simulink model "HDLLTE"  (R2017b)
settings: Solver=FixedStepDiscrete  StartTime=0.0  StopTime=simParams.stopTime  RelTol=1e-3
InitFcn:
  | simParams = hdlcoder_lteofdm_modDetectref_init;
  | simParams = hdlcoder_lteofdm_modDetecthdl_init(simParams);
StopFcn:
  | hdlcoder_lteofdm_modDetect_analyze;
undefined symbols (not defined in the file): fft_size
libraries: hdlsllib x29, simulink x22, simulink_need_slupdate x13, dspxfrm3 x2, commchan3 x1, dspmlti4 x1, commrflib2 x1, hdlcodermisc x1, dspsigops x1, dspmathops x1, dspsrcs4 x1
(part 2 of 3)

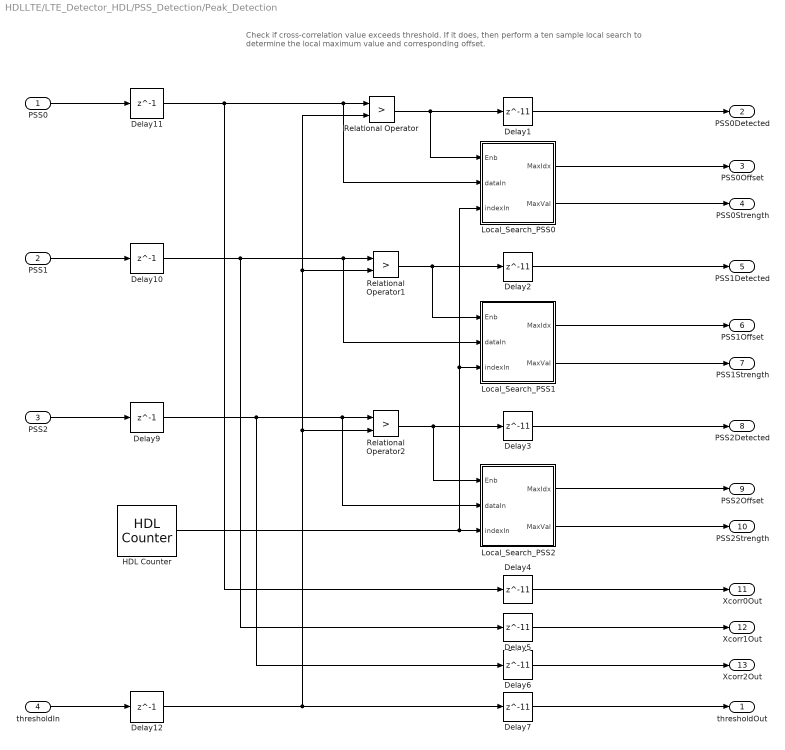
== system HDLLTE/LTE_Detector_HDL/PSS_Detection/Peak_Detection ==
  note: Check if cross-correlation value exceeds threshold. If it does, then perform a ten sample local search to determine the local maximum value and corresponding offset.
  PSS0 : Inport
  PSS1 : Inport  Port=2
  PSS2 : Inport  Port=3
  thresholdIn : Inport  Port=4
  Delay{1..7} (7 alike) : Delay  DelayLength=11  InitialCondition=0
  Delay{9..12} (4 alike) : Delay  DelayLength=1  InitialCondition=0  UseCircularBuffer=on
  HDL Counter : hdlsllib/Sources/HDL Counter  CountType=Count limited  CountInit=0  CountStep=1  CountMax=19199  CountFromType=Initial value  CountFrom=0  CountResetPort=off  CountLoadPort=off  CountEnbPort=off  CountDirPort=off  CountDataType=Unsigned  CountWordLen=ceil(log2(19199))  CountFracLen=0  CountSampTime=simParams.TsRx
      settings: SourceProductBaseCode=HD
  Local_Search_PSS0 : Subsystem
  Local_Search_PSS1 : Subsystem
  Local_Search_PSS2 : Subsystem
  Relational Operator : RelationalOperator  Operator=>  OutDataTypeStr=boolean  RndMeth=Nearest
  Relational Operator1 : RelationalOperator  Operator=>  OutDataTypeStr=boolean  RndMeth=Nearest
  Relational Operator2 : RelationalOperator  Operator=>  OutDataTypeStr=boolean  RndMeth=Nearest
  thresholdOut : Outport  InitialOutput=0
  PSS0Detected : Outport  Port=2
  PSS0Offset : Outport  Port=3
  PSS0Strength : Outport  Port=4
  PSS1Detected : Outport  Port=5
  PSS1Offset : Outport  Port=6
  PSS1Strength : Outport  Port=7
  PSS2Detected : Outport  Port=8
  PSS2Offset : Outport  Port=9
  PSS2Strength : Outport  Port=10
  Xcorr0Out : Outport  Port=11  InitialOutput=0
  Xcorr1Out : Outport  Port=12  InitialOutput=0
  Xcorr2Out : Outport  Port=13  InitialOutput=0
  wires:
  thresholdIn/1 -> Delay12/1
  PSS2/1 -> Delay9/1
  PSS1/1 -> Delay10/1
  Relational Operator/1 -> Delay1/1, Local_Search_PSS0/1(Enb)
  Relational Operator1/1 -> Local_Search_PSS1/1(Enb), Delay2/1
  Relational Operator2/1 -> Local_Search_PSS2/1(Enb), Delay3/1
  PSS0/1 -> Delay11/1
  Local_Search_PSS0/1(MaxIdx) -> PSS0Offset/1
  Local_Search_PSS0/2(MaxVal) -> PSS0Strength/1
  Local_Search_PSS1/1(MaxIdx) -> PSS1Offset/1
  Local_Search_PSS1/2(MaxVal) -> PSS1Strength/1
  Local_Search_PSS2/1(MaxIdx) -> PSS2Offset/1
  Local_Search_PSS2/2(MaxVal) -> PSS2Strength/1
  Delay1/1 -> PSS0Detected/1
  Delay2/1 -> PSS1Detected/1
  Delay3/1 -> PSS2Detected/1
  Delay4/1 -> Xcorr0Out/1
  Delay5/1 -> Xcorr1Out/1
  Delay6/1 -> Xcorr2Out/1
  Delay7/1 -> thresholdOut/1
  HDL Counter/1 -> Local_Search_PSS2/3(indexIn), Local_Search_PSS1/3(indexIn), Local_Search_PSS0/3(indexIn)
  Delay9/1 -> Delay6/1, Local_Search_PSS2/2(dataIn), Relational Operator2/1
  Delay10/1 -> Delay5/1, Local_Search_PSS1/2(dataIn), Relational Operator1/1
  Delay11/1 -> Local_Search_PSS0/2(dataIn), Relational Operator/1, Delay4/1
  Delay12/1 -> Relational Operator/2, Relational Operator1/2, Relational Operator2/2, Delay7/1

== system HDLLTE/LTE_Detector_HDL/SSS_Detection/SSS_Dot_Product ==
  note: Accumulate
  note: Reset register after all 63 samples have been processed
  note: Only final sample from accumulator is valid
  note: Multiply dataIn by seqIn:
      | since seqIn is always either -1 or 1, use a gain of -1 and a switch to invert dataIn when seqIn = -1.
  dataIn : Inport
  validIn : Inport  Port=2
  seqIn : Inport  Port=3
  reset : Inport  Port=4
  Add : Sum  OutDataTypeStr=Inherit: Same as first input
  Compare To Zero1 : simulink/Logic and Bit Operations/Compare To Zero  relop=<  OutDataTypeStr=boolean
  Data Type Conversion : DataTypeConversion  OutDataTypeStr=fixdt(1,24,10)
  Data Type Conversion1 : DataTypeConversion  OutDataTypeStr=fixdt(1,18,4)  RndMeth=Round
  Delay Reset : Subsystem
  Delay1 : Delay  DelayLength=1  InitialCondition=0
  Delay2 : Delay  DelayLength=4  InitialCondition=0
  Delay3 : Delay  InitialCondition=0
  Delay5 : Delay  DelayLength=1  InitialCondition=0
  Gain : Gain  Gain=-1  OutDataTypeStr=Inherit: Same as input
  Magnitude Squared 0 : Subsystem
  real1 : Switch  Criteria=u2 ~= 0
  validOut : Outport  InitialOutput=0
  SSSDotProd : Outport  Port=2  InitialOutput=0
  wires:
  Delay2/1 -> validOut/1
  Delay3/1 -> Delay2/1, Delay Reset/3(R)
  Delay5/1 -> Delay Reset/2(E)
  Add/1 -> Delay Reset/1(u)
  validIn/1 -> Delay5/1
  Delay1/1 -> Data Type Conversion/1
  Magnitude Squared 0/1(Magnitude^2) -> SSSDotProd/1
  reset/1 -> Delay3/1
  Delay Reset/1(y) -> Add/2, Data Type Conversion1/1
  Data Type Conversion/1 -> Add/1
  real1/1 -> Delay1/1
  dataIn/1 -> Gain/1, real1/3
  Gain/1 -> real1/1
  seqIn/1 -> Compare To Zero1/1
  Compare To Zero1/1 -> real1/2
  Data Type Conversion1/1 -> Magnitude Squared 0/1(dataIn)

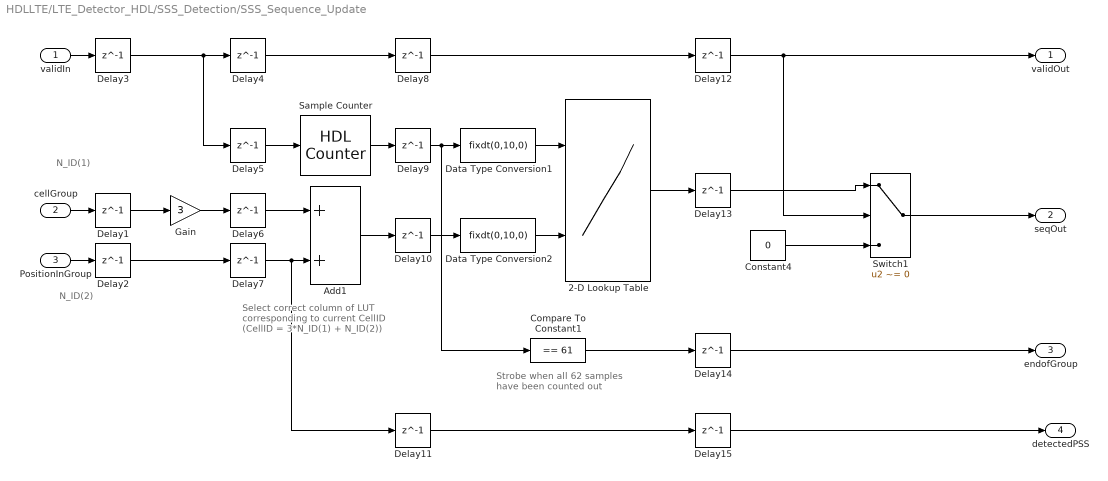
== system HDLLTE/LTE_Detector_HDL/SSS_Detection/SSS_Sequence_Update ==
  note: N_ID(2)
  note: Select correct column of LUT
      | corresponding to current CellID
      | (CellID = 3*N_ID(1) + N_ID(2))
  note: N_ID(1)
  note: Strobe when all 62 samples
      | have been counted out
  validIn : Inport
  cellGroup : Inport  Port=2
  PositionInGroup : Inport  Port=3
  2-D Lookup Table : Lookup_n-D  BreakpointsForDimension1=[0:size(simParams.possibleSSS,1)-1]  BreakpointsForDimension2=[0:size(simParams.possibleSSS,2)-1]  IndexSearchMethod=Evenly spaced points  Table=real(simParams.possibleSSS)  TableDataTypeStr=fixdt(1,2,0)  InterpMethod=Flat  DiagnosticForOutOfRangeInput=Error  InternalRulePriority=Speed  OutDataTypeStr=fixdt(1,2,0)  RndMeth=Simplest  InputSameDT=on
  Add1 : Sum  OutDataTypeStr=Inherit: Same as first input
  Compare To Constant1 : simulink/Logic and Bit Operations/Compare To Constant  relop===  const=61  OutDataTypeStr=boolean
  Constant4 : Constant  Value=0  OutDataTypeStr=fixdt(1,2,0)  SampleTime=simParams.TsRx
  Data Type Conversion1 : DataTypeConversion  OutDataTypeStr=fixdt(0,10,0)
  Data Type Conversion2 : DataTypeConversion  OutDataTypeStr=fixdt(0,10,0)
  Delay{1..15} (15 alike) : Delay  DelayLength=1  InitialCondition=0
  Gain : Gain  Gain=3  OutDataTypeStr=fixdt(0,10,0)
  Sample Counter : hdlsllib/Sources/HDL Counter  CountType=Count limited  CountInit=0  CountStep=1  CountMax=61  CountFromType=Initial value  CountFrom=0  CountResetPort=off  CountLoadPort=off  CountEnbPort=on  CountDirPort=off  CountDataType=Unsigned  CountWordLen=ceil(log2(61))  CountFracLen=0  CountSampTime=1
      settings: SourceProductBaseCode=HD
  Switch1 : Switch  Criteria=u2 ~= 0
  validOut : Outport  InitialOutput=0
  seqOut : Outport  Port=2  InitialOutput=0
  endofGroup : Outport  Port=3  InitialOutput=0
  detectedPSS : Outport  Port=4  InitialOutput=0
  wires:
  Constant4/1 -> Switch1/3
  Data Type Conversion1/1 -> 2-D Lookup Table/1
  Data Type Conversion2/1 -> 2-D Lookup Table/2
  2-D Lookup Table/1 -> Delay13/1
  Compare To Constant1/1 -> Delay14/1
  cellGroup/1 -> Delay1/1
  Gain/1 -> Delay6/1
  validIn/1 -> Delay3/1
  Sample Counter/1 -> Delay9/1
  Add1/1 -> Delay10/1
  PositionInGroup/1 -> Delay2/1
  Delay3/1 -> Delay4/1, Delay5/1
  Delay1/1 -> Gain/1
  Delay2/1 -> Delay7/1
  Delay4/1 -> Delay8/1
  Delay5/1 -> Sample Counter/1
  Delay6/1 -> Add1/1
  Delay7/1 -> Delay11/1, Add1/2
  Delay8/1 -> Delay12/1
  Delay9/1 -> Data Type Conversion1/1, Compare To Constant1/1
  Delay10/1 -> Data Type Conversion2/1
  Delay11/1 -> Delay15/1
  Delay12/1 -> validOut/1, Switch1/2
  Delay13/1 -> Switch1/1
  Switch1/1 -> seqOut/1
  Delay14/1 -> endofGroup/1
  Delay15/1 -> detectedPSS/1

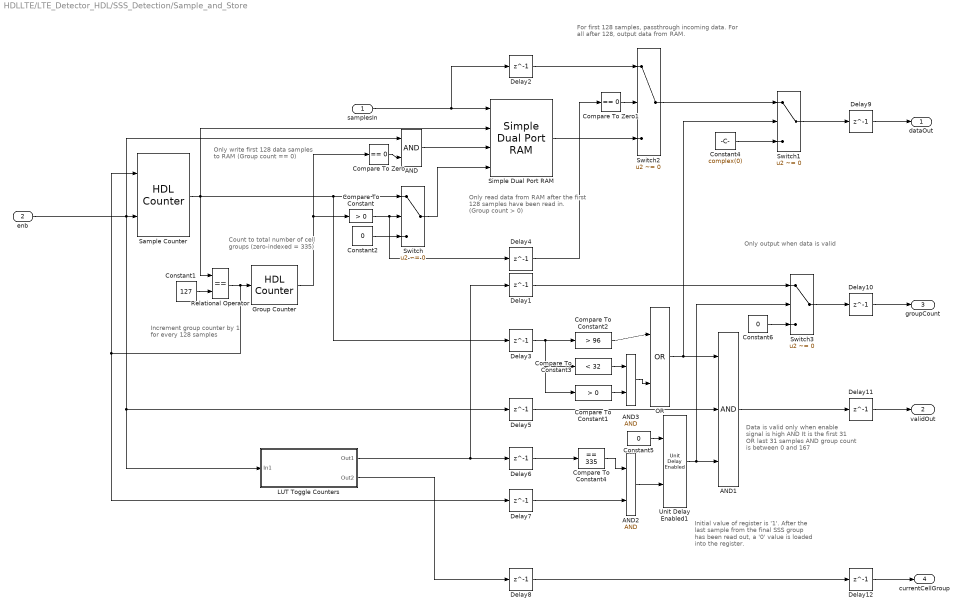
== system HDLLTE/LTE_Detector_HDL/SSS_Detection/Sample_and_Store ==
  note: Count to total number of
      | cell groups
      | (zero-indexed = 335)
  note: For first 128 samples, passthrough incoming data.
      | For all after 128, output data from RAM.
  note: Data is valid only when enable
      | signal is high AND It is the first
      | 31 OR last 31 samples AND
      | group count is between 0 and 167
  note: Only read data from RAM after the
      | first 128 samples have been read in.
      | (Group count > 0)
  note: Only write first 128 data samples
      | to RAM (Group count == 0)
  note: Increment group counter by 1
      | for every 128 samples
  note: Initial value of register is '1'.
      | After the last sample from the
      | final SSS group has been read out,
      | a '0' value is loaded into the register.
  note: Only output when data is valid
  samplesIn : Inport
  enb : Inport  Port=2
  AND : Logic  IconShape=distinctive  AllPortsSameDT=off  OutDataTypeStr=boolean
  AND1 : Logic  Inputs=3  IconShape=distinctive  AllPortsSameDT=off  OutDataTypeStr=boolean
  AND2 : Logic  IconShape=distinctive  AllPortsSameDT=off  OutDataTypeStr=boolean
  AND3 : Logic  IconShape=distinctive  AllPortsSameDT=off  OutDataTypeStr=boolean
  Compare To Constant : simulink/Logic and Bit Operations/Compare To Constant  relop=>  const=0  OutDataTypeStr=boolean
  Compare To Constant1 : simulink/Logic and Bit Operations/Compare To Constant  relop=>  const=0  OutDataTypeStr=boolean
  Compare To Constant2 : simulink/Logic and Bit Operations/Compare To Constant  relop=>  const=96  OutDataTypeStr=boolean
  Compare To Constant3 : simulink/Logic and Bit Operations/Compare To Constant  relop=<  const=32  OutDataTypeStr=boolean
  Compare To Constant4 : simulink/Logic and Bit Operations/Compare To Constant  relop===  const=335  OutDataTypeStr=boolean
  Compare To Zero : simulink/Logic and Bit Operations/Compare To Zero  relop===  OutDataTypeStr=boolean
  Compare To Zero1 : simulink/Logic and Bit Operations/Compare To Zero  relop===  OutDataTypeStr=boolean
  Constant1 : Constant  Value=127  OutDataTypeStr=fixdt(0,8,0)  SampleTime=simParams.TsRx
  Constant2 : Constant  Value=0  OutDataTypeStr=fixdt(0,7,0)  SampleTime=simParams.TsRx
  Constant4 : Constant  Value=complex(0)  OutDataTypeStr=Inherit: Inherit via back propagation  SampleTime=simParams.TsRx
  Constant5 : Constant  Value=0  OutDataTypeStr=boolean  SampleTime=simParams.TsRx
  Constant6 : Constant  Value=0  OutDataTypeStr=fixdt(0,9,0)  SampleTime=simParams.TsRx
  Delay{1..12} (12 alike) : Delay  DelayLength=1  InitialCondition=0
  Group Counter : hdlsllib/Sources/HDL Counter  CountType=Count limited  CountInit=0  CountStep=1  CountMax=335  CountFromType=Initial value  CountFrom=0  CountResetPort=off  CountLoadPort=off  CountEnbPort=on  CountDirPort=off  CountDataType=Unsigned  CountWordLen=ceil(log2(335))  CountFracLen=0  CountSampTime=1
      settings: SourceProductBaseCode=HD
  LUT Toggle Counters : Subsystem
  OR : Logic  Operator=OR  IconShape=distinctive  AllPortsSameDT=off  OutDataTypeStr=boolean
  Relational Operator : RelationalOperator  Operator===  OutDataTypeStr=boolean  RndMeth=Nearest
  Sample Counter : hdlsllib/Sources/HDL Counter  CountType=Count limited  CountInit=0  CountStep=1  CountMax=127  CountFromType=Initial value  CountFrom=0  CountResetPort=on  CountLoadPort=off  CountEnbPort=on  CountDirPort=off  CountDataType=Unsigned  CountWordLen=log2(128)  CountFracLen=0  CountSampTime=1
      settings: SourceProductBaseCode=HD
  Simple Dual Port RAM : hdlsllib/HDL RAMs/Simple Dual Port RAM  ram_size=7
      settings: SourceProductName=HDL Coder  SourceProductBaseCode=HD
  Switch : Switch  Criteria=u2 ~= 0
  Switch1 : Switch  Criteria=u2 ~= 0  InputSameDT=on
  Switch2 : Switch  Criteria=u2 ~= 0
  Switch3 : Switch  Criteria=u2 ~= 0
  Unit Delay Enabled1 : simulink_need_slupdate/Unit Delay Enabled  vinit=1  tsamp=-1
      settings: SourceProductName=Simulink  SourceProductBaseCode=SL
  dataOut : Outport
  validOut : Outport  Port=2
  groupCount : Outport  Port=3
  currentCellGroup : Outport  Port=4
  wires:
  Compare To Constant1/1 -> AND3/2
  Compare To Constant3/1 -> AND3/1
  AND3/1 -> OR/2
  Constant6/1 -> Switch3/3
  Delay7/1 -> AND2/2
  Unit Delay Enabled1/1 -> AND1/3, Switch3/2
  AND2/1 -> Unit Delay Enabled1/2
  Constant5/1 -> Unit Delay Enabled1/1
  samplesIn/1 -> Simple Dual Port RAM/1, Delay2/1
  Delay5/1 -> AND1/2
  Delay4/1 -> Compare To Zero1/1
  Delay3/1 -> Compare To Constant3/1, Compare To Constant1/1, Compare To Constant2/1
  Delay2/1 -> Switch2/1
  Switch2/1 -> Switch1/1
  Simple Dual Port RAM/1 -> Switch2/3
  Compare To Zero1/1 -> Switch2/2
  Constant4/1 -> Switch1/3
  OR/1 -> AND1/1, Switch1/2
  Compare To Constant2/1 -> OR/1
  Constant2/1 -> Switch/3
  Switch/1 -> Simple Dual Port RAM/4
  Compare To Zero/1 -> AND/2
  Compare To Constant/1 -> Switch/2, Delay4/1
  AND/1 -> Simple Dual Port RAM/3
  Constant1/1 -> Relational Operator/2
  enb/1 -> AND/1, Delay5/1, LUT Toggle Counters/1(In1), Sample Counter/2
  Group Counter/1 -> Compare To Constant/1, Compare To Zero/1
  Sample Counter/1 -> Switch/1, Delay3/1, Relational Operator/1, Simple Dual Port RAM/2
  Delay1/1 -> Switch3/1
  LUT Toggle Counters/1(Out1) -> Delay6/1, Delay1/1
  Delay6/1 -> Compare To Constant4/1
  Compare To Constant4/1 -> AND2/1
  Relational Operator/1 -> Group Counter/1, Delay7/1, Sample Counter/1
  Switch1/1 -> Delay9/1
  Switch3/1 -> Delay10/1
  AND1/1 -> Delay11/1
  LUT Toggle Counters/2(Out2) -> Delay8/1
  Delay8/1 -> Delay12/1
  Delay9/1 -> dataOut/1
  Delay10/1 -> groupCount/1
  Delay11/1 -> validOut/1
  Delay12/1 -> currentCellGroup/1

== system HDLLTE/LTE_Modulator_HDL/CP_Extension_Windowing/Compute_CP_Pass_Through_Index ==
  note: Select cyclic prefix length
  note: increment the OFDM symbol counter
      | which goes from 0 to 6
  note: Detect switch from 1 to 0 on validIn.
      | This indicates the end of an OFDM symbol
  validIn : Inport
  Add : Sum  Inputs=+-  OutDataTypeStr=uint16
  Add1 : Sum  OutDataTypeStr=uint16
  Compare To Zero : simulink/Logic and Bit Operations/Compare To Zero  relop===  OutDataTypeStr=boolean
  Constant4 : Constant  Value=simParams.nFFT  VectorParams1D=off  OutDataTypeStr=uint16  SampleTime=simParams.TsTx
  Delay1 : Delay  DelayLength=1  InitialCondition=0  InputProcessing=Columns as channels (frame based)
  Length of first CP : Constant  Value=160*(simParams.nFFT/2048)+simParams.windowing  OutDataTypeStr=uint16  SampleTime=simParams.TsTx
  Length of other CPs : Constant  Value=144*(simParams.nFFT/2048)+simParams.windowing  OutDataTypeStr=uint16  SampleTime=simParams.TsTx
  Logical Operator : Logic  IconShape=distinctive  AllPortsSameDT=off  OutDataTypeStr=boolean
  Logical Operator1 : Logic  Operator=NOT  IconShape=distinctive  AllPortsSameDT=off  OutDataTypeStr=boolean
  OFDM Symbol Counter : hdlsllib/Sources/HDL Counter  CountType=Count limited  CountInit=0  CountStep=1  CountMax=6  CountFromType=Initial value  CountFrom=0  CountResetPort=off  CountLoadPort=off  CountEnbPort=on  CountDirPort=off  CountDataType=Unsigned  CountWordLen=3  CountFracLen=0  CountSampTime=1
      settings: SourceProductBaseCode=HD
  Switch : Switch  Criteria=u2 ~= 0
  window length : Constant  Value=simParams.windowing  OutDataTypeStr=uint16  SampleTime=simParams.TsTx
  fftMinusCPandWindow : Outport
  fftMinusCP : Outport  Port=2
  wires:
  Logical Operator1/1 -> Logical Operator/1
  Length of first CP/1 -> Switch/1
  Length of other CPs/1 -> Switch/3
  OFDM Symbol Counter/1 -> Compare To Zero/1
  Compare To Zero/1 -> Switch/2
  Switch/1 -> Add/2
  validIn/1 -> Delay1/1, Logical Operator1/1
  Delay1/1 -> Logical Operator/2
  Logical Operator/1 -> OFDM Symbol Counter/1
  Constant4/1 -> Add/1
  window length/1 -> Add1/2
  Add1/1 -> fftMinusCP/1
  Add/1 -> fftMinusCPandWindow/1, Add1/1

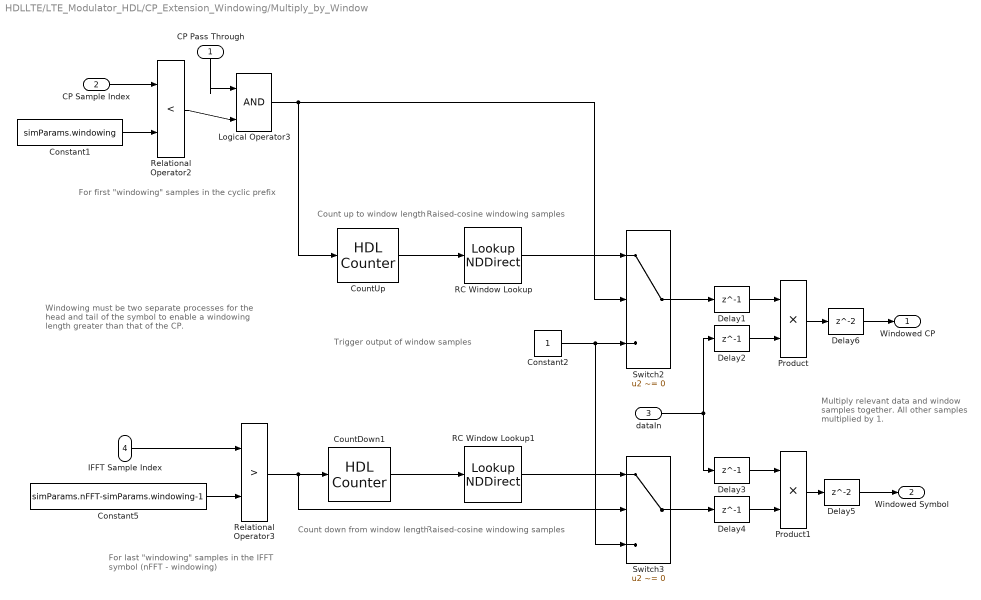
== system HDLLTE/LTE_Modulator_HDL/CP_Extension_Windowing/Multiply_by_Window ==
  note: Windowing must be two separate processes for the
      | head and tail of the symbol to enable a
      | windowing length greater than that of the CP.
  note: Multiply relevant data and window
      | samples together. All other samples
      | multiplied by 1.
  note: Count up to window length
  note: Trigger output of window samples
  note: For last "windowing" samples in the IFFT
      | symbol (nFFT - windowing)
  note: For first "windowing" samples in the cyclic prefix
  note: Raised-cosine windowing samples
  note: Count down from window length
  note: Raised-cosine windowing samples
  CP Pass Through : Inport
  CP Sample Index : Inport  Port=2
  dataIn : Inport  Port=3
  IFFT Sample Index : Inport  Port=4
  Constant1 : Constant  Value=simParams.windowing  OutDataTypeStr=uint16  SampleTime=simParams.TsTx
  Constant2 : Constant  OutDataTypeStr=fixdt(1,16,15)  SampleTime=simParams.TsTx
  Constant5 : Constant  Value=simParams.nFFT-simParams.windowing-1  OutDataTypeStr=int16  SampleTime=simParams.TsTx
  CountDown1 : hdlsllib/Sources/HDL Counter  CountType=Count limited  CountInit=simParams.LUTwindowing-1  CountStep=-1  CountMax=0  CountFromType=Initial value  CountFrom=simParams.LUTwindowing-1  CountResetPort=off  CountLoadPort=off  CountEnbPort=on  CountDirPort=off  CountDataType=Unsigned  CountWordLen=8  CountFracLen=0  CountSampTime=1
      settings: SourceProductBaseCode=HD
  CountUp : hdlsllib/Sources/HDL Counter  CountType=Count limited  CountInit=0  CountStep=1  CountMax=simParams.LUTwindowing-1  CountFromType=Initial value  CountFrom=0  CountResetPort=off  CountLoadPort=off  CountEnbPort=on  CountDirPort=off  CountDataType=Unsigned  CountWordLen=8  CountFracLen=0  CountSampTime=1
      settings: SourceProductBaseCode=HD
  Delay{1..4} (4 alike) : Delay  DelayLength=1  InitialCondition=0  InputProcessing=Columns as channels (frame based)
  Delay5 : Delay  InitialCondition=0  InputProcessing=Columns as channels (frame based)
  Delay6 : Delay  InitialCondition=0  InputProcessing=Columns as channels (frame based)
  Logical Operator3 : Logic  IconShape=distinctive  AllPortsSameDT=off  OutDataTypeStr=boolean
  Product : Product  OutDataTypeStr=Inherit: Inherit via back propagation
  Product1 : Product  OutDataTypeStr=Inherit: Inherit via back propagation
  RC Window Lookup : LookupNDDirect  NumberOfTableDimensions=1  Table=simParams.RCWindow  DiagnosticForOutOfRangeInput=Error  TableDataTypeStr=fixdt(1,16,15)
  RC Window Lookup1 : LookupNDDirect  NumberOfTableDimensions=1  Table=simParams.RCWindow  DiagnosticForOutOfRangeInput=Error  TableDataTypeStr=fixdt(1,16,15)
  Relational Operator2 : RelationalOperator  Operator=<  OutDataTypeStr=boolean  RndMeth=Nearest
  Relational Operator3 : RelationalOperator  Operator=>  OutDataTypeStr=boolean  RndMeth=Nearest
  Switch2 : Switch  Criteria=u2 ~= 0
  Switch3 : Switch  Criteria=u2 ~= 0
  Windowed CP : Outport
  Windowed Symbol : Outport  Port=2
  wires:
  Product/1 -> Delay6/1
  RC Window Lookup/1 -> Switch2/1
  CP Sample Index/1 -> Relational Operator2/1
  Constant1/1 -> Relational Operator2/2
  Relational Operator2/1 -> Logical Operator3/2
  Constant5/1 -> Relational Operator3/2
  Switch2/1 -> Delay1/1
  Product1/1 -> Delay5/1
  Switch3/1 -> Delay4/1
  Constant2/1 -> Switch3/3, Switch2/3
  IFFT Sample Index/1 -> Relational Operator3/1
  CP Pass Through/1 -> Logical Operator3/1
  RC Window Lookup1/1 -> Switch3/1
  CountUp/1 -> RC Window Lookup/1
  CountDown1/1 -> RC Window Lookup1/1
  Relational Operator3/1 -> Switch3/2, CountDown1/1
  Logical Operator3/1 -> Switch2/2, CountUp/1
  dataIn/1 -> Delay3/1, Delay2/1
  Delay1/1 -> Product/1
  Delay4/1 -> Product1/2
  Delay2/1 -> Product/2
  Delay3/1 -> Product1/1
  Delay5/1 -> Windowed Symbol/1
  Delay6/1 -> Windowed CP/1

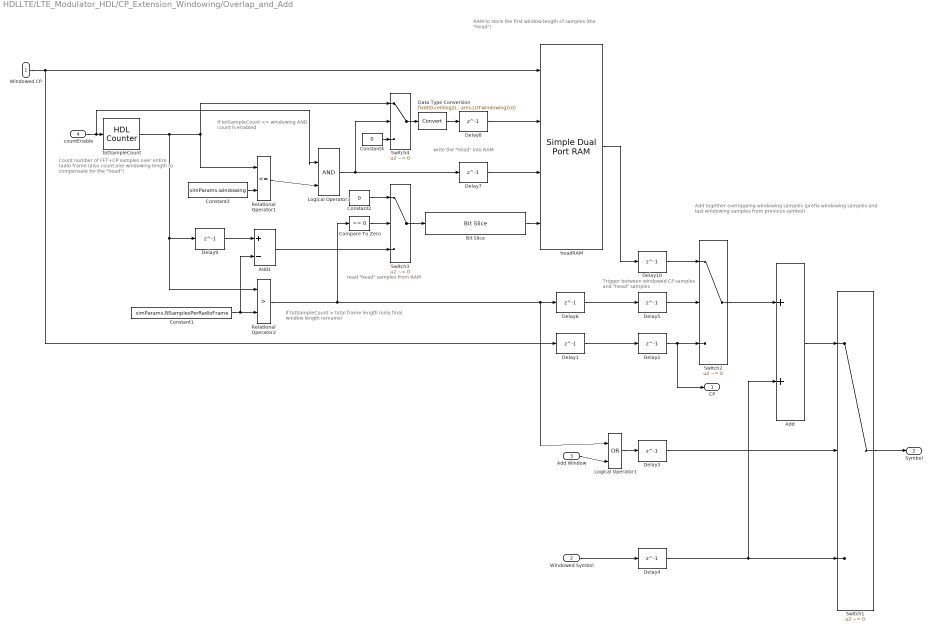
== system HDLLTE/LTE_Modulator_HDL/CP_Extension_Windowing/Overlap_and_Add ==
  note: Trigger between windowed CP samples
      | and "head" samples
  note: read "head" samples from RAM
  note: write the "head" into RAM
  note: If totSampleCount <= windowing
      | AND count is enabled
  note: if totSampleCount > total frame length
      | (only final window length remains)
  note: Add together overlapping windowing samples
      | (prefix windowing samples and last windowing samples
      | from previous symbol)
  note: RAM to store the first window length of
      | samples (the "head")
  note: Count number of FFT+CP samples
      | over entire radio frame
      | (also count one windowing length
      | to compensate for the "head")
  Windowed CP : Inport
  Windowed Symbol : Inport  Port=2
  Add Window : Inport  Port=3
  countEnable : Inport  Port=4
  Add : Sum  OutDataTypeStr=Inherit: Inherit via back propagation
  Add1 : Sum  Inputs=+-
  Bit Slice : hdlsllib/Logic and Bit Operations/Bit Slice  lidx=ceil(log2(simParams.LUTwindowing))-1  ridx=0
  Compare To Zero : simulink/Logic and Bit Operations/Compare To Zero  relop===  OutDataTypeStr=boolean
  Constant1 : Constant  Value=simParams.NSamplesPerRadioFrame  OutDataTypeStr=fixdt(0,ceil(log2(simParams.NSamplesPerRadioFrame+1)),0)  SampleTime=simParams.TsTx
  Constant2 : Constant  Value=0  OutDataTypeStr=fixdt(0,ceil(log2(simParams.LUTwindowing)),0)  SampleTime=simParams.TsTx
  Constant3 : Constant  Value=simParams.windowing  OutDataTypeStr=fixdt(0,ceil(log2(simParams.LUTwindowing)),0)  SampleTime=simParams.TsTx
  Constant4 : Constant  Value=0  OutDataTypeStr=fixdt(0,ceil(log2(simParams.LUTwindowing)),0)  SampleTime=simParams.TsTx
  Data Type Conversion : DataTypeConversion  OutDataTypeStr=fixdt(0,ceil(log2(simParams.LUTwindowing)),0)
  Delay{1..10} (10 alike) : Delay  DelayLength=1  InitialCondition=0  InputProcessing=Columns as channels (frame based)
  Logical Operator1 : Logic  Operator=OR  IconShape=distinctive  AllPortsSameDT=off  OutDataTypeStr=boolean
  Logical Operator3 : Logic  IconShape=distinctive  AllPortsSameDT=off  OutDataTypeStr=boolean
  Relational Operator1 : RelationalOperator  Operator=<=  OutDataTypeStr=boolean  RndMeth=Nearest
  Relational Operator2 : RelationalOperator  Operator=>  OutDataTypeStr=boolean  RndMeth=Nearest
  Switch{1..4} (4 alike) : Switch  Criteria=u2 ~= 0
  headRAM : hdlsllib/HDL RAMs/Simple Dual Port RAM  ram_size=ceil(log2(simParams.LUTwindowing))
      settings: SourceProductName=HDL Coder  SourceProductBaseCode=HD
  totSampleCount : hdlsllib/Sources/HDL Counter  CountType=Count limited  CountInit=0  CountStep=1  CountMax=simParams.NSamplesPerRadioFrame+simParams.windowing+1  CountFromType=Initial value  CountFrom=0  CountResetPort=off  CountLoadPort=off  CountEnbPort=on  CountDirPort=off  CountDataType=Unsigned  CountWordLen=ceil(log2(simParams.NSamplesPerRadioFrame+simParams.windowing+1))  CountFracLen=0  CountSampTime=1
      settings: SourceProductBaseCode=HD
  CP : Outport
  Symbol : Outport  Port=2
  wires:
  totSampleCount/1 -> Relational Operator2/1, Delay9/1, Switch4/1, Relational Operator1/1
  Constant3/1 -> Relational Operator1/2
  Data Type Conversion/1 -> Delay8/1
  Add/1 -> Switch1/1
  Logical Operator3/1 -> Delay7/1, Switch4/2
  Relational Operator1/1 -> Logical Operator3/2
  Logical Operator1/1 -> Delay3/1
  Delay1/1 -> Delay2/1
  Switch2/1 -> Add/1
  Add1/1 -> Switch3/3
  Switch1/1 -> Symbol/1
  Relational Operator2/1 -> Compare To Zero/1, Delay6/1, Logical Operator1/1
  Constant1/1 -> Add1/2, Relational Operator2/2
  headRAM/1 -> Delay10/1
  Constant2/1 -> Switch3/1
  Compare To Zero/1 -> Switch3/2
  Windowed Symbol/1 -> Delay4/1
  Add Window/1 -> Logical Operator1/2
  countEnable/1 -> Logical Operator3/1, totSampleCount/1
  Delay2/1 -> CP/1, Switch2/3
  Delay3/1 -> Switch1/2
  Delay4/1 -> Add/2, Switch1/3
  Delay5/1 -> Switch2/2
  Switch4/1 -> Data Type Conversion/1
  Constant4/1 -> Switch4/3
  Windowed CP/1 -> headRAM/1, Delay1/1
  Delay7/1 -> headRAM/3
  Delay8/1 -> headRAM/2
  Delay9/1 -> Add1/1
  Delay10/1 -> Switch2/1
  Switch3/1 -> Bit Slice/1
  Bit Slice/1 -> headRAM/4
  Delay6/1 -> Delay5/1

== system HDLLTE/LTE_Modulator_HDL/FFT_Shift/Compute_Read_Address ==
  note: XOR with FFT size/2 performs the fftshift on the address
      | as it flips the MSB of the index in the IFFT,
      | while XOR with FFT size flips the ping/pong
  note: select enough bits to represent 2*fft_size addresses
  note: Ping/Pong Read Address so reading from half of BlockRAM not being written to.
  note: Load Read Ptr with 0
      | and count up to fft_size  to read out data
  note: When rdEnable goes high toggle offset for Ping/Pong buffer for Read Ptr.
      | Make sure REAd and WRITE Ptr are not in same section of Ping/Pong
  note: Initial counter output is FFT size setting the counter enable to '0'.
      | When the rdEnable signal comes in, the value of 0 is loaded into
      | the counter accumulator AND output. This triggers the
      | enable signal to '1', and the counter will count up to FFT size
      | before the enable goes to '0', where the counter will remain until
      | the next load signal arrives.
  note: Alternates between outputting a '0' and '1'
      | each time the read signal is toggled high.
  rdEnable : Inport
  Bit Slice : hdlsllib/Logic and Bit Operations/Bit Slice  lidx=log2(simParams.nFFT)  ridx=0
  Bitwise Operator1 : simulink/Logic and Bit Operations/Bitwise Operator  logicop=XOR  UseBitMask=off  NumInputPorts=2  BitMask=fft_size/2  BitMaskRealWorld=Stored Integer
  Compare To Constant4 : simulink/Logic and Bit Operations/Compare To Constant  relop=<  const=simParams.nFFT  OutDataTypeStr=boolean
  Constant3 : Constant  Value=simParams.nFFT/2  OutDataTypeStr=uint16  SampleTime=simParams.TsTx
  Constant4 : Constant  Value=simParams.nFFT+simParams.nFFT/2  OutDataTypeStr=uint16  SampleTime=simParams.TsTx
  Constant6 : Constant  Value=0  OutDataTypeStr=uint16  SampleTime=simParams.TsTx
  Delay3 : Delay  DelayLength=1
  HDL Counter1 : hdlsllib/Sources/HDL Counter  CountType=Free running  CountInit=simParams.nFFT  CountStep=1  CountMax=10  CountFromType=Initial value  CountFrom=simParams.nFFT  CountResetPort=off  CountLoadPort=on  CountEnbPort=on  CountDirPort=off  CountDataType=Unsigned  CountWordLen=16  CountFracLen=0  CountSampTime=1
      settings: SourceProductBaseCode=HD
  Not : Logic  Operator=NOT  IconShape=distinctive  AllPortsSameDT=off  OutDataTypeStr=boolean
  Switch : Switch  Criteria=u2 ~= 0  Threshold=384
  Switch2 : Switch  Criteria=u2 ~= 0  Threshold=384
  rdAddr : Outport
  rdValid : Outport  Port=2
  wires:
  HDL Counter1/1 -> Compare To Constant4/1, Bitwise Operator1/1
  Compare To Constant4/1 -> HDL Counter1/3, rdValid/1
  Switch2/1 -> Delay3/1, Switch/2
  Delay3/1 -> Switch2/3, Not/1
  Not/1 -> Switch2/1
  Constant6/1 -> HDL Counter1/2
  rdEnable/1 -> HDL Counter1/1, Switch2/2
  Bit Slice/1 -> rdAddr/1
  Constant4/1 -> Switch/3
  Constant3/1 -> Switch/1
  Switch/1 -> Bitwise Operator1/2
  Bitwise Operator1/1 -> Bit Slice/1

== system HDLLTE/LTE_Modulator_HDL/OFDM_Symbol_Mapping/IFFT_Subcarrier_Counter ==
  note: Reset signal takes one clock cycle to register.
      | So reset should be triggered when count value
      | equals nFFT+CPlength-1 .
      | Hence use of nFFT-1.
  note: CP length selection.
      | 7 OFDM symbols per slot. The first symbol in the slot
      | has a longer CP length.
  note: Count until output is equal to FFT size + current CP.
      | When equal, resets bin counter and increments symbol counter.
  note: First sample values are < 0, and are reserved for the CP, and the bin count is held at nFFT . Otherwise outputs in the range of
      | 0 -> nFFT .
  Add : Sum
  Compare To Zero : simulink/Logic and Bit Operations/Compare To Zero  relop===  OutDataTypeStr=boolean
  Compare To Zero1 : simulink/Logic and Bit Operations/Compare To Zero  relop=>=  OutDataTypeStr=boolean
  FFT Size : Constant  Value=simParams.nFFT-1  OutDataTypeStr=fixdt(0,ceil(log2(simParams.nFFT)),0)  SampleTime=simParams.TsTx
  FFT Size1 : Constant  Value=simParams.nFFT  OutDataTypeStr=fixdt(0,ceil(log2(simParams.nFFT))+2,0)  SampleTime=simParams.TsTx
  HDL Counter : hdlsllib/Sources/HDL Counter  CountType=Count limited  CountInit=0  CountStep=1  CountMax=6  CountFromType=Initial value  CountFrom=0  CountResetPort=off  CountLoadPort=off  CountEnbPort=on  CountDirPort=off  CountDataType=Unsigned  CountWordLen=3  CountFracLen=0  CountSampTime=1
      settings: SourceProductBaseCode=HD
  HDL Counter2 : hdlsllib/Sources/HDL Counter  CountType=Free running  CountInit=0  CountStep=1  CountMax=6  CountFromType=Initial value  CountFrom=0  CountResetPort=on  CountLoadPort=off  CountEnbPort=off  CountDirPort=off  CountDataType=Unsigned  CountWordLen=ceil(log2(simParams.nFFT))+1  CountFracLen=0  CountSampTime=1
      settings: SourceProductBaseCode=HD
  Length of first CP : Constant  Value=160*(simParams.nFFT/2048)  OutDataTypeStr=fixdt(0,ceil(log2(simParams.nFFT)),0)  SampleTime=simParams.TsTx
  Length of other CPs : Constant  Value=144*(simParams.nFFT/2048)  OutDataTypeStr=fixdt(0,ceil(log2(simParams.nFFT)),0)  SampleTime=simParams.TsTx
  Relational Operator : RelationalOperator  Operator===  OutDataTypeStr=boolean  RndMeth=Nearest
  Subtract : Sum  Inputs=+-  OutDataTypeStr=fixdt(1,ceil(log2(simParams.nFFT))+2,0)
  Switch : Switch  Criteria=u2 ~= 0
  Switch1 : Switch  Criteria=u2 ~= 0
  IFFT subcarrier : Outport
  wires:
  Compare To Zero/1 -> Switch/2
  HDL Counter2/1 -> Subtract/1, Relational Operator/1  "Count"
  Switch/1 -> Subtract/2, Add/2
  [INCREMENT_SYMBOL] -> HDL Counter/1
  Compare To Zero1/1 -> Switch1/2
  Switch1/1 -> IFFT subcarrier/1
  Add/1 -> Relational Operator/2
  FFT Size1/1 -> Switch1/3
  Relational Operator/1 -> HDL Counter2/1, [INCREMENT_SYMBOL]
  HDL Counter/1 -> Compare To Zero/1
  Length of other CPs/1 -> Switch/3
  Subtract/1 -> Compare To Zero1/1, Switch1/1
  Length of first CP/1 -> Switch/1
  FFT Size/1 -> Add/1

== system HDLLTE/LTE_Detector_HDL/Frequency_Estimation/Cyclic_Prefix_Correlator/Moving_Average ==
  note: Use a comb filter followed by an integrator
      | to implement an efficient 9-tab moving average.
  dataIn : Inport
  Add : Sum  Inputs=-+  AccumDataTypeStr=fixdt(1,27,23)
  Add1 : Sum  AccumDataTypeStr=fixdt(1,27,23)
  Delay1 : Delay  DelayLength=8  InitialCondition=0
  Delay10 : Delay  DelayLength=1  InitialCondition=0  UseCircularBuffer=on
  Delay2 : Delay  DelayLength=1  InitialCondition=0  UseCircularBuffer=on
  Delay3 : Delay  DelayLength=1  InitialCondition=0  UseCircularBuffer=on
  Gain : Gain  Gain=1/8  OutDataTypeStr=fixdt(1,24,23)
  dataOut : Outport
  wires:
  Add/1 -> Delay10/1
  dataIn/1 -> Add/2, Delay1/1
  Delay1/1 -> Add/1
  Add1/1 -> Delay2/1
  Delay10/1 -> Add1/2
  Delay2/1 -> Gain/1, Add1/1
  Gain/1 -> Delay3/1
  Delay3/1 -> dataOut/1

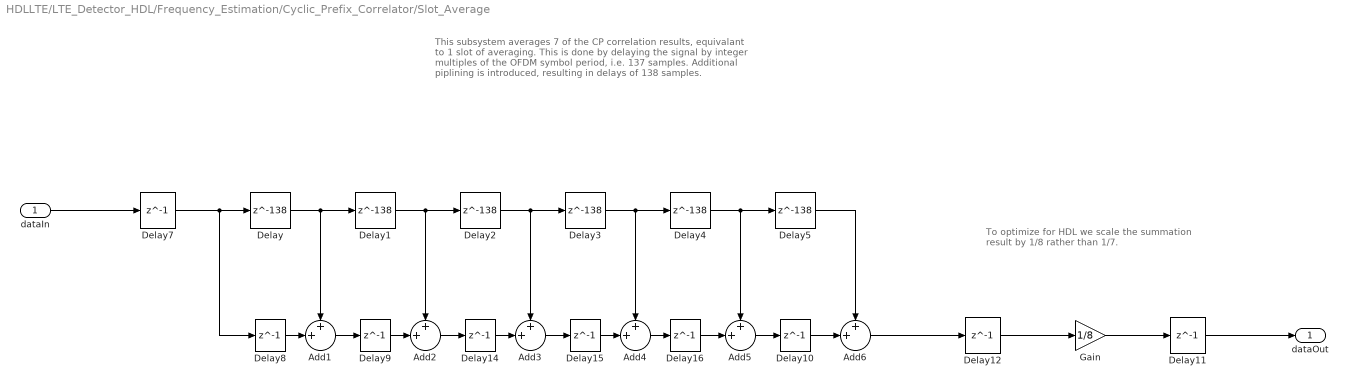
== system HDLLTE/LTE_Detector_HDL/Frequency_Estimation/Cyclic_Prefix_Correlator/Slot_Average ==
  note: This subsystem averages 7 of the CP correlation results, equivalant to 1 slot of averaging. This is done by delaying the signal by integer multiples of the OFDM symbol period, i.e. 137 samples.
      |
      | Additional piplining is introduced, resulting in delays of 138 samples.
  note: To optimize for HDL we scale the summation result by 1/8 rather than 1/7.
  dataIn : Inport
  Add1 : Sum  Inputs=++|  AccumDataTypeStr=fixdt(1,28,23)
  Add2 : Sum  Inputs=++|  AccumDataTypeStr=fixdt(1,29,23)
  Add3 : Sum  Inputs=++|  OutDataTypeStr=fixdt(1,29,23)
  Add4 : Sum  Inputs=++|  AccumDataTypeStr=fixdt(1,29,23)
  Add5 : Sum  Inputs=++|  AccumDataTypeStr=fixdt(1,30,23)
  Add6 : Sum  Inputs=++|  AccumDataTypeStr=fixdt(1,30,23)
  Delay{,1..5} (6 alike) : Delay  DelayLength=138  InitialCondition=0
  Delay{7..12,14..16} (9 alike) : Delay  DelayLength=1  InitialCondition=0  UseCircularBuffer=on
  Gain : Gain  Gain=1/8  OutDataTypeStr=fixdt(1,24,23)
  dataOut : Outport
  wires:
  Delay4/1 -> Delay5/1, Add5/1
  Delay/1 -> Delay1/1, Add1/1
  Add1/1 -> Delay9/1
  Delay1/1 -> Delay2/1, Add2/1
  Delay3/1 -> Delay4/1, Add4/1
  Delay2/1 -> Delay3/1, Add3/1
  dataIn/1 -> Delay7/1
  Add2/1 -> Delay14/1
  Add3/1 -> Delay15/1
  Add4/1 -> Delay16/1
  Add5/1 -> Delay10/1
  Delay5/1 -> Add6/1
  Add6/1 -> Delay12/1
  Delay7/1 -> Delay8/1, Delay/1
  Delay8/1 -> Add1/2
  Delay9/1 -> Add2/2
  Delay14/1 -> Add3/2
  Delay15/1 -> Add4/2
  Delay16/1 -> Add5/2
  Delay10/1 -> Add6/2
  Delay12/1 -> Gain/1
  Gain/1 -> Delay11/1
  Delay11/1 -> dataOut/1

== system HDLLTE/LTE_Detector_HDL/PSS_Detection/Cross_Correlation/Averaging_Filter ==
  datIn : Inport
  Add : Sum  Inputs=-+  AccumDataTypeStr=fixdt(1,32,23)  OutDataTypeStr=Inherit: Same as accumulator
  Add1 : Sum  AccumDataTypeStr=fixdt(1,32,23)  OutDataTypeStr=Inherit: Same as accumulator
  Delay1 : Delay  DelayLength=128  InitialCondition=0
  Delay2 : Delay  DelayLength=1  InitialCondition=0  UseCircularBuffer=on
  Delay3 : Delay  DelayLength=1  InitialCondition=0  UseCircularBuffer=on
  Gain : Gain  Gain=2^-7  OutDataTypeStr=fixdt(1,25,23)
  thresholdOut : Outport
  wires:
  Delay3/1 -> Add1/2
  Add1/1 -> Delay2/1
  Add/1 -> Delay3/1
  Delay2/1 -> Gain/1, Add1/1
  Delay1/1 -> Add/1
  datIn/1 -> Add/2, Delay1/1
  Gain/1 -> thresholdOut/1

== system HDLLTE/LTE_Detector_HDL/PSS_Detection/Cross_Correlation/Magnitude_Squared ==
  dataIn : Inport
  Add : Sum  OutDataTypeStr=Inherit: Same as accumulator
  Complex to Real-Imag : ComplexToRealImag
  Data Type Conversion : DataTypeConversion  OutDataTypeStr=fixdt(1,25,23)  RndMeth=Round
  Delay1 : Delay  InitialCondition=0
  Delay2 : Delay  InitialCondition=0
  Delay3 : Delay  DelayLength=1  InitialCondition=0
  Delay4 : Delay  DelayLength=1  InitialCondition=0
  Delay5 : Delay  DelayLength=1  InitialCondition=0
  Product1 : Product
  Product4 : Product
  Magnitude^2 : Outport
  wires:
  Delay4/1 -> Data Type Conversion/1
  Delay2/1 -> Add/1
  Delay1/1 -> Add/2
  Delay3/1 -> Complex to Real-Imag/1
  dataIn/1 -> Delay3/1
  Product4/1 -> Delay2/1
  Complex to Real-Imag/2 -> Product1/1, Product1/2
  Complex to Real-Imag/1 -> Product4/1, Product4/2
  Add/1 -> Delay4/1
  Product1/1 -> Delay1/1
  Delay5/1 -> Magnitude^2/1
  Data Type Conversion/1 -> Delay5/1

== system HDLLTE/LTE_Detector_HDL/PSS_Detection/Cross_Correlation/Magnitude_Squared_0 ==
  dataIn : Inport
  Add : Sum  OutDataTypeStr=Inherit: Same as accumulator
  Complex to Real-Imag : ComplexToRealImag
  Delay1 : Delay  InitialCondition=0
  Delay2 : Delay  InitialCondition=0
  Delay3 : Delay  DelayLength=1  InitialCondition=0
  Delay4 : Delay  InitialCondition=0
  Product4 : Product
  Product5 : Product
  Magnitude^2 : Outport
  wires:
  Delay4/1 -> Magnitude^2/1
  Delay2/1 -> Add/2
  Delay1/1 -> Add/1
  Delay3/1 -> Complex to Real-Imag/1
  dataIn/1 -> Delay3/1
  Product4/1 -> Delay1/1
  Complex to Real-Imag/2 -> Product5/1, Product5/2
  Complex to Real-Imag/1 -> Product4/1, Product4/2
  Add/1 -> Delay4/1
  Product5/1 -> Delay2/1

== system HDLLTE/LTE_Detector_HDL/PSS_Detection/Cross_Correlation/Magnitude_Squared_1 ==
  dataIn : Inport
  Add : Sum  OutDataTypeStr=Inherit: Same as accumulator
  Complex to Real-Imag : ComplexToRealImag
  Delay1 : Delay  InitialCondition=0
  Delay2 : Delay  InitialCondition=0
  Delay3 : Delay  DelayLength=1  InitialCondition=0
  Delay4 : Delay  InitialCondition=0
  Product4 : Product
  Product5 : Product
  Magnitude^2 : Outport
  wires:
  Delay4/1 -> Magnitude^2/1
  Delay2/1 -> Add/2
  Delay1/1 -> Add/1
  Delay3/1 -> Complex to Real-Imag/1
  dataIn/1 -> Delay3/1
  Product4/1 -> Delay1/1
  Complex to Real-Imag/2 -> Product5/1, Product5/2
  Complex to Real-Imag/1 -> Product4/1, Product4/2
  Add/1 -> Delay4/1
  Product5/1 -> Delay2/1

== system HDLLTE/LTE_Detector_HDL/PSS_Detection/Cross_Correlation/Magnitude_Squared_2 ==
  dataIn : Inport
  Add : Sum  OutDataTypeStr=Inherit: Same as accumulator
  Complex to Real-Imag : ComplexToRealImag
  Delay1 : Delay  InitialCondition=0
  Delay2 : Delay  InitialCondition=0
  Delay3 : Delay  DelayLength=1  InitialCondition=0
  Delay4 : Delay  InitialCondition=0
  Product4 : Product
  Product5 : Product
  Magnitude^2 : Outport
  wires:
  Delay4/1 -> Magnitude^2/1
  Delay2/1 -> Add/2
  Delay1/1 -> Add/1
  Delay3/1 -> Complex to Real-Imag/1
  dataIn/1 -> Delay3/1
  Product4/1 -> Delay1/1
  Complex to Real-Imag/2 -> Product5/1, Product5/2
  Complex to Real-Imag/1 -> Product4/1, Product4/2
  Add/1 -> Delay4/1
  Product5/1 -> Delay2/1

== system HDLLTE/LTE_Detector_HDL/PSS_Detection/Cross_Correlation/PSSXCorr0 ==
  note: B
  note: A
  dataIn : Inport
  C : DiscreteFir  Coefficients=real(simParams.PSS(:,PSSIdx)')  CoefDataTypeStr=fixdt(1,18)
  C+D : DiscreteFir  Coefficients=real(simParams.PSS(:,PSSIdx)') + imag(simParams.PSS(:,PSSIdx)')  CoefDataTypeStr=fixdt(1,18)
  C-D : DiscreteFir  Coefficients=real(simParams.PSS(:,PSSIdx)') - imag(simParams.PSS(:,PSSIdx)')  CoefDataTypeStr=fixdt(1,18)
  Complex to Real-Imag1 : ComplexToRealImag
  Data Type Conversion : DataTypeConversion  OutDataTypeStr=fixdt(1,16,10)  RndMeth=Round
  Delay{1..5,10,14} (7 alike) : Delay  DelayLength=1  InitialCondition=0
  Real-Imag to Complex1 : RealImagToComplex
  Sum2 : Sum  Inputs=-+
  Sum3 : Sum  Inputs=-+
  Sum4 : Sum
  dataOut : Outport
  wires:
  dataIn/1 -> Delay1/1
  Real-Imag to Complex1/1 -> Data Type Conversion/1
  Sum2/1 -> Delay5/1
  Complex to Real-Imag1/1 -> Delay14/1, Sum2/1
  Complex to Real-Imag1/2 -> Delay10/1, Sum2/2
  C/1 -> Sum4/1, Sum3/1
  C-D/1 -> Sum3/2
  C+D/1 -> Sum4/2
  Sum3/1 -> Delay4/1
  Sum4/1 -> Delay3/1
  Delay1/1 -> Complex to Real-Imag1/1
  Delay2/1 -> dataOut/1
  Delay3/1 -> Real-Imag to Complex1/2
  Delay4/1 -> Real-Imag to Complex1/1
  Delay5/1 -> C/1
  Delay10/1 -> C-D/1
  Delay14/1 -> C+D/1
  Data Type Conversion/1 -> Delay2/1

== system HDLLTE/LTE_Detector_HDL/PSS_Detection/Cross_Correlation/PSSXCorr1 ==
  note: B
  note: A
  dataIn : Inport
  C : DiscreteFir  Coefficients=real(simParams.PSS(:,PSSIdx)')  CoefDataTypeStr=fixdt(1,18)
  C+D : DiscreteFir  Coefficients=real(simParams.PSS(:,PSSIdx)') + imag(simParams.PSS(:,PSSIdx)')  CoefDataTypeStr=fixdt(1,18)
  C-D : DiscreteFir  Coefficients=real(simParams.PSS(:,PSSIdx)') - imag(simParams.PSS(:,PSSIdx)')  CoefDataTypeStr=fixdt(1,18)
  Complex to Real-Imag1 : ComplexToRealImag
  Data Type Conversion : DataTypeConversion  OutDataTypeStr=fixdt(1,16,10)  RndMeth=Round
  Delay{1..5,10,14} (7 alike) : Delay  DelayLength=1  InitialCondition=0
  Real-Imag to Complex1 : RealImagToComplex
  Sum2 : Sum  Inputs=-+
  Sum3 : Sum  Inputs=-+
  Sum4 : Sum
  dataOut : Outport
  wires:
  dataIn/1 -> Delay1/1
  Real-Imag to Complex1/1 -> Data Type Conversion/1
  Sum2/1 -> Delay5/1
  Complex to Real-Imag1/1 -> Delay14/1, Sum2/1
  Complex to Real-Imag1/2 -> Delay10/1, Sum2/2
  C/1 -> Sum4/1, Sum3/1
  C-D/1 -> Sum3/2
  C+D/1 -> Sum4/2
  Sum3/1 -> Delay4/1
  Sum4/1 -> Delay3/1
  Delay1/1 -> Complex to Real-Imag1/1
  Delay2/1 -> dataOut/1
  Delay3/1 -> Real-Imag to Complex1/2
  Delay4/1 -> Real-Imag to Complex1/1
  Delay5/1 -> C/1
  Delay10/1 -> C-D/1
  Delay14/1 -> C+D/1
  Data Type Conversion/1 -> Delay2/1

== system HDLLTE/LTE_Detector_HDL/PSS_Detection/Cross_Correlation/PSSXCorr2 ==
  note: B
  note: A
  dataIn : Inport
  C : DiscreteFir  Coefficients=real(simParams.PSS(:,PSSIdx)')  CoefDataTypeStr=fixdt(1,18)
  C+D : DiscreteFir  Coefficients=real(simParams.PSS(:,PSSIdx)') + imag(simParams.PSS(:,PSSIdx)')  CoefDataTypeStr=fixdt(1,18)
  C-D : DiscreteFir  Coefficients=real(simParams.PSS(:,PSSIdx)') - imag(simParams.PSS(:,PSSIdx)')  CoefDataTypeStr=fixdt(1,18)
  Complex to Real-Imag1 : ComplexToRealImag
  Data Type Conversion : DataTypeConversion  OutDataTypeStr=fixdt(1,16,10)  RndMeth=Round
  Delay{1..5,10,14} (7 alike) : Delay  DelayLength=1  InitialCondition=0
  Real-Imag to Complex1 : RealImagToComplex
  Sum2 : Sum  Inputs=-+
  Sum3 : Sum  Inputs=-+
  Sum4 : Sum
  dataOut : Outport
  wires:
  dataIn/1 -> Delay1/1
  Real-Imag to Complex1/1 -> Data Type Conversion/1
  Sum2/1 -> Delay5/1
  Complex to Real-Imag1/1 -> Delay14/1, Sum2/1
  Complex to Real-Imag1/2 -> Delay10/1, Sum2/2
  C/1 -> Sum4/1, Sum3/1
  C-D/1 -> Sum3/2
  C+D/1 -> Sum4/2
  Sum3/1 -> Delay4/1
  Sum4/1 -> Delay3/1
  Delay1/1 -> Complex to Real-Imag1/1
  Delay2/1 -> dataOut/1
  Delay3/1 -> Real-Imag to Complex1/2
  Delay4/1 -> Real-Imag to Complex1/1
  Delay5/1 -> C/1
  Delay10/1 -> C-D/1
  Delay14/1 -> C+D/1
  Data Type Conversion/1 -> Delay2/1

== system HDLLTE/LTE_Detector_HDL/PSS_Detection/Peak_Detection/Local_Search_PSS0 ==
  note: Generate 10 sample enable signal
  Enb : Inport
  dataIn : Inport  Port=2
  indexIn : Inport  Port=3
  Add : Sum  AccumDataTypeStr=fixdt(0,15,0)
  Constant1 : Constant  Value=0  VectorParams1D=off  OutDataTypeStr=fixdt(0,22,20)  SampleTime=simParams.TsRx
  Constant2 : Constant  Value=11  VectorParams1D=off  OutDataTypeStr=fixdt(0,4,0)  SampleTime=simParams.TsRx
  Delay1 : Delay  DelayLength=11  InitialCondition=0
  Delay2 : Delay  DelayLength=1  InitialCondition=0
  Delay21 : Delay  DelayLength=1  InitialCondition=0  InputProcessing=Columns as channels (frame based)
  Delay3 : Delay  DelayLength=1  InitialCondition=0  InputProcessing=Columns as channels (frame based)
  HDL Counter : hdlsllib/Sources/HDL Counter  CountType=Count limited  CountInit=1  CountStep=1  CountMax=11  CountFromType=Initial value  CountFrom=1  CountResetPort=off  CountLoadPort=off  CountEnbPort=on  CountDirPort=off  CountDataType=Unsigned  CountWordLen=4  CountFracLen=0  CountSampTime=1
      settings: SourceProductBaseCode=HD
  Logical Operator2 : Logic  Operator=OR  AllPortsSameDT=off  OutDataTypeStr=boolean
  Relational Operator1 : RelationalOperator  Operator=<  OutDataTypeStr=boolean  RndMeth=Nearest
  Relational Operator2 : RelationalOperator  Operator=>  OutDataTypeStr=boolean  RndMeth=Nearest
  Switch1 : Switch  Criteria=u2 ~= 0  Threshold=384
  maximum : Subsystem
  MaxIdx : Outport
  MaxVal : Outport  Port=2
  wires:
  Enb/1 -> Logical Operator2/1
  maximum/1(MaxVal) -> Delay21/1
  dataIn/1 -> Delay2/1
  maximum/2(MaxIdx) -> Relational Operator2/1, Add/1
  Add/1 -> Delay3/1
  Relational Operator2/1 -> Switch1/2
  indexIn/1 -> Delay1/1
  Constant1/1 -> Switch1/3, Relational Operator2/2
  Switch1/1 -> Add/2
  Delay1/1 -> Switch1/1
  Constant2/1 -> Relational Operator1/2
  Logical Operator2/1 -> HDL Counter/1
  Relational Operator1/1 -> maximum/2(Enb), Logical Operator2/2
  Delay2/1 -> maximum/1(dataIn)
  Delay21/1 -> MaxVal/1
  Delay3/1 -> MaxIdx/1
  HDL Counter/1 -> Relational Operator1/1

== system HDLLTE/LTE_Detector_HDL/PSS_Detection/Peak_Detection/Local_Search_PSS1 ==
  note: Generate 10 sample enable signal
  Enb : Inport
  dataIn : Inport  Port=2
  indexIn : Inport  Port=3
  Add : Sum  AccumDataTypeStr=fixdt(0,15,0)
  Constant1 : Constant  Value=0  VectorParams1D=off  OutDataTypeStr=fixdt(0,22,20)  SampleTime=simParams.TsRx
  Constant2 : Constant  Value=11  VectorParams1D=off  OutDataTypeStr=fixdt(0,4,0)  SampleTime=simParams.TsRx
  Delay1 : Delay  DelayLength=11  InitialCondition=0
  Delay2 : Delay  DelayLength=1  InitialCondition=0
  Delay21 : Delay  DelayLength=1  InitialCondition=0  InputProcessing=Columns as channels (frame based)
  Delay3 : Delay  DelayLength=1  InitialCondition=0  InputProcessing=Columns as channels (frame based)
  HDL Counter : hdlsllib/Sources/HDL Counter  CountType=Count limited  CountInit=1  CountStep=1  CountMax=11  CountFromType=Initial value  CountFrom=1  CountResetPort=off  CountLoadPort=off  CountEnbPort=on  CountDirPort=off  CountDataType=Unsigned  CountWordLen=4  CountFracLen=0  CountSampTime=1
      settings: SourceProductBaseCode=HD
  Logical Operator2 : Logic  Operator=OR  AllPortsSameDT=off  OutDataTypeStr=boolean
  Relational Operator1 : RelationalOperator  Operator=<  OutDataTypeStr=boolean  RndMeth=Nearest
  Relational Operator2 : RelationalOperator  Operator=>  OutDataTypeStr=boolean  RndMeth=Nearest
  Switch1 : Switch  Criteria=u2 ~= 0  Threshold=384
  maximum : Subsystem
  MaxIdx : Outport
  MaxVal : Outport  Port=2
  wires:
  HDL Counter/1 -> Relational Operator1/1
  Delay3/1 -> MaxIdx/1
  Delay21/1 -> MaxVal/1
  Delay2/1 -> maximum/1(dataIn)
  Relational Operator1/1 -> Logical Operator2/2, maximum/2(Enb)
  Logical Operator2/1 -> HDL Counter/1
  Constant2/1 -> Relational Operator1/2
  Delay1/1 -> Switch1/1
  Switch1/1 -> Add/2
  Constant1/1 -> Relational Operator2/2, Switch1/3
  indexIn/1 -> Delay1/1
  Relational Operator2/1 -> Switch1/2
  Add/1 -> Delay3/1
  maximum/2(MaxIdx) -> Add/1, Relational Operator2/1
  dataIn/1 -> Delay2/1
  maximum/1(MaxVal) -> Delay21/1
  Enb/1 -> Logical Operator2/1

== system HDLLTE/LTE_Detector_HDL/PSS_Detection/Peak_Detection/Local_Search_PSS2 ==
  note: Generate 10 sample enable signal
  Enb : Inport
  dataIn : Inport  Port=2
  indexIn : Inport  Port=3
  Add : Sum  AccumDataTypeStr=fixdt(0,15,0)
  Constant1 : Constant  Value=0  VectorParams1D=off  OutDataTypeStr=fixdt(0,22,20)  SampleTime=simParams.TsRx
  Constant2 : Constant  Value=11  VectorParams1D=off  OutDataTypeStr=fixdt(0,4,0)  SampleTime=simParams.TsRx
  Delay1 : Delay  DelayLength=11  InitialCondition=0
  Delay2 : Delay  DelayLength=1  InitialCondition=0
  Delay21 : Delay  DelayLength=1  InitialCondition=0  InputProcessing=Columns as channels (frame based)
  Delay3 : Delay  DelayLength=1  InitialCondition=0  InputProcessing=Columns as channels (frame based)
  HDL Counter : hdlsllib/Sources/HDL Counter  CountType=Count limited  CountInit=1  CountStep=1  CountMax=11  CountFromType=Initial value  CountFrom=1  CountResetPort=off  CountLoadPort=off  CountEnbPort=on  CountDirPort=off  CountDataType=Unsigned  CountWordLen=4  CountFracLen=0  CountSampTime=1
      settings: SourceProductBaseCode=HD
  Logical Operator2 : Logic  Operator=OR  AllPortsSameDT=off  OutDataTypeStr=boolean
  Relational Operator1 : RelationalOperator  Operator=<  OutDataTypeStr=boolean  RndMeth=Nearest
  Relational Operator2 : RelationalOperator  Operator=>  OutDataTypeStr=boolean  RndMeth=Nearest
  Switch1 : Switch  Criteria=u2 ~= 0  Threshold=384
  maximum : Subsystem
  MaxIdx : Outport
  MaxVal : Outport  Port=2
  wires:
  Enb/1 -> Logical Operator2/1
  maximum/1(MaxVal) -> Delay21/1
  dataIn/1 -> Delay2/1
  maximum/2(MaxIdx) -> Relational Operator2/1, Add/1
  Add/1 -> Delay3/1
  Relational Operator2/1 -> Switch1/2
  indexIn/1 -> Delay1/1
  Constant1/1 -> Switch1/3, Relational Operator2/2
  Switch1/1 -> Add/2
  Delay1/1 -> Switch1/1
  Constant2/1 -> Relational Operator1/2
  Logical Operator2/1 -> HDL Counter/1
  Relational Operator1/1 -> maximum/2(Enb), Logical Operator2/2
  Delay2/1 -> maximum/1(dataIn)
  Delay21/1 -> MaxVal/1
  Delay3/1 -> MaxIdx/1
  HDL Counter/1 -> Relational Operator1/1

== system HDLLTE/LTE_Detector_HDL/SSS_Detection/SSS_Dot_Product/Delay Reset ==
  note: Enable
  u : Inport
  E : Inport  Port=2
  R : Inport  Port=3
  Enable : Switch  Criteria=u2 > Threshold  OutDataTypeStr=Inherit: Inherit via back propagation  ZeroCross=off
  Reset Delay : Subsystem
  y : Outport
  wires:
  R/1 -> Reset Delay/2(R1)
  Enable/1 -> Reset Delay/1(u1)
  u/1 -> Enable/1
  Reset Delay/1(Out1) -> y/1, Enable/3
  E/1 -> Enable/2

== system HDLLTE/LTE_Detector_HDL/SSS_Detection/SSS_Dot_Product/Magnitude Squared 0 ==
  dataIn : Inport
  Add : Sum  OutDataTypeStr=Inherit: Same as first input
  Complex to Real-Imag : ComplexToRealImag
  Delay1 : Delay  InitialCondition=0
  Delay2 : Delay  InitialCondition=0
  Delay3 : Delay  DelayLength=1  InitialCondition=0
  Delay4 : Delay  InitialCondition=0
  Product4 : Product
  Product5 : Product
  Magnitude^2 : Outport
  wires:
  Delay4/1 -> Magnitude^2/1
  Delay2/1 -> Add/2
  Delay1/1 -> Add/1
  Delay3/1 -> Complex to Real-Imag/1
  dataIn/1 -> Delay3/1
  Product4/1 -> Delay1/1
  Complex to Real-Imag/2 -> Product5/1, Product5/2
  Complex to Real-Imag/1 -> Product4/1, Product4/2
  Add/1 -> Delay4/1
  Product5/1 -> Delay2/1

== system HDLLTE/LTE_Detector_HDL/SSS_Detection/Sample_and_Store/LUT Toggle Counters ==
  In1 : Inport
  Compare To Constant4 : simulink/Logic and Bit Operations/Compare To Constant  relop===  const=255  OutDataTypeStr=boolean
  Compare To Constant5 : simulink/Logic and Bit Operations/Compare To Constant  relop=<  const=128  OutDataTypeStr=boolean
  Index SubFrame 0 : hdlsllib/Sources/HDL Counter  CountType=Count limited  CountInit=0  CountStep=1  CountMax=167  CountFromType=Initial value  CountFrom=0  CountResetPort=off  CountLoadPort=off  CountEnbPort=on  CountDirPort=off  CountDataType=Unsigned  CountWordLen=ceil(log2(167))  CountFracLen=0  CountSampTime=1
      settings: SourceProductBaseCode=HD
  Index SubFrame 5 : hdlsllib/Sources/HDL Counter  CountType=Count limited  CountInit=168  CountStep=1  CountMax=335  CountFromType=Initial value  CountFrom=168  CountResetPort=off  CountLoadPort=off  CountEnbPort=on  CountDirPort=off  CountDataType=Unsigned  CountWordLen=ceil(log2(335))  CountFracLen=0  CountSampTime=1
      settings: SourceProductBaseCode=HD
  Sample Counter1 : hdlsllib/Sources/HDL Counter  CountType=Count limited  CountInit=0  CountStep=1  CountMax=255  CountFromType=Initial value  CountFrom=0  CountResetPort=off  CountLoadPort=off  CountEnbPort=on  CountDirPort=off  CountDataType=Unsigned  CountWordLen=ceil(log2(255))  CountFracLen=0  CountSampTime=1
      settings: SourceProductBaseCode=HD
  Switch4 : Switch  Criteria=u2 ~= 0
  Out1 : Outport
  Out2 : Outport  Port=2
  wires:
  Index SubFrame 5/1 -> Switch4/3
  Compare To Constant4/1 -> Index SubFrame 5/1, Index SubFrame 0/1
  Sample Counter1/1 -> Compare To Constant5/1, Compare To Constant4/1
  Compare To Constant5/1 -> Switch4/2
  Index SubFrame 0/1 -> Out2/1, Switch4/1
  In1/1 -> Sample Counter1/1
  Switch4/1 -> Out1/1
